simulink model "dof3_vehicle_tests"  (R2019a)
settings: Solver=VariableStepAuto  StartTime=0.0  StopTime=15.0  RelTol=1e-3
libraries: autolibshared x1, simulink x1
settings Model: Creator=Fernando VM  LastModifiedBy=fvall
settings DataIOCC: ReturnWorkspaceOutputs=off
settings DebuggingCC: ArithmeticOperatorsInVariantConditions=warning

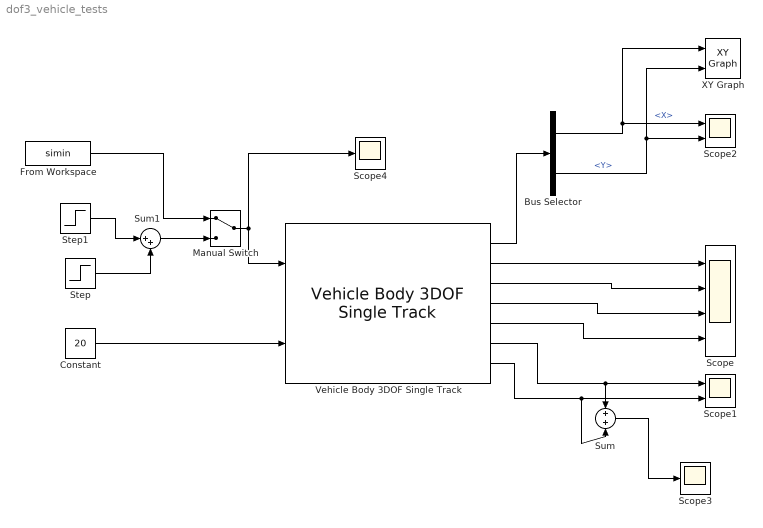
== system dof3_vehicle_tests ==
  Bus Selector : BusSelector  OutputSignals=InertFrm.Cg.Disp.X,InertFrm.Cg.Disp.Y
  Constant : Constant  Value=20
  From Workspace : FromWorkspace  VariableName=simin  SampleTime=0
  Manual Switch : ManualSwitch
  Scope : Scope  NumInputPorts=4
  Scope1 : Scope  NumInputPorts=2
  Scope2 : Scope  NumInputPorts=2
  Scope3 : Scope
  Scope4 : Scope
  Step : Step  After=0.05  SampleTime=0
  Step1 : Step  Time=3.5  After=-0.1  SampleTime=0
  Sum : Sum
  Sum1 : Sum  Inputs=|++
  Vehicle Body 3DOF Single Track : autolibshared/Vehicle Body 3DOF Single Track  trackMode=Single (bicycle)  inputMode=External longitudinal velocity  frontSteerMode=on  rearSteerMode=off  windMode=off  muMode=off  extFMode=off  extMMode=off  extXo=off  extpsio=off  extxdoto=off  extro=off  extYo=off  extTamb=off  extydoto=off  aMode=2  NF=2  NR=2  m=2000  a=1.4  b=1.6  h=0.35  X_o=0  xdot_o=20  CalphaMode=off  sigmaMode=on  d=0  w=[1.4,1.4]  Cy_f=12e3  Cy_r=11e3  sigma_f=.1  sigma_r=.1  alpha_f_brk=[-.1 .1]  Cy_f_data=[-9e3 9e3]  alpha_r_brk=[-.1 .1]  Cy_r_data=[-9e3 9e3]  Y_o=0  ydot_o=0  Izz=4000  psi_o=0  r_o=0  Af=2  Cd=.3  Cl=.1  Cpm=.1  beta_w=[0:0.01:0.3]  Cs=[0:0.03:0.9]  Cym=[0:0.01:0.3]  Pabs=101325  Tair=273  g=9.81  mu=1  xdot_tol=.01  Fznom=5000  Fxtire_sat=7e4  Fytire_sat=7e4  longOff=0  latOff=0  vertOff=0  wrapAng=off
      settings: SourceProductName=Powertrain Blockset  SourceProductBaseCode=PW
  XY Graph : simulink/Sinks/XY Graph  xmin=0  xmax=300  ymin=0  ymax=10  st=-1
  wires:
  Constant/1 -> Vehicle Body 3DOF Single Track/2
  Vehicle Body 3DOF Single Track/3 -> Scope/2
  Vehicle Body 3DOF Single Track/2 -> Scope/1
  Vehicle Body 3DOF Single Track/4 -> Scope/3
  Vehicle Body 3DOF Single Track/5 -> Scope/4
  Vehicle Body 3DOF Single Track/1 -> Bus Selector/1
  Bus Selector/1 -> Scope2/1, XY Graph/1  "<X>"
  Bus Selector/2 -> Scope2/2, XY Graph/2  "<Y>"
  Vehicle Body 3DOF Single Track/6 -> Scope1/1, Sum/1
  Vehicle Body 3DOF Single Track/7 -> Sum/2, Scope1/2
  Sum/1 -> Scope3/1
  Step/1 -> Sum1/2
  Step1/1 -> Sum1/1
  Manual Switch/1 -> Vehicle Body 3DOF Single Track/1, Scope4/1
  Sum1/1 -> Manual Switch/2
  From Workspace/1 -> Manual Switch/1
